simulink model "adc_sim"  (R2017a)
settings: Solver=VariableStepAuto  StartTime=0.0  StopTime=1  FixedStep=0.1e-6  RelTol=1e-3
settings Model: Creator=Andrei Purcarus  LastModifiedBy=Andrei Purcarus

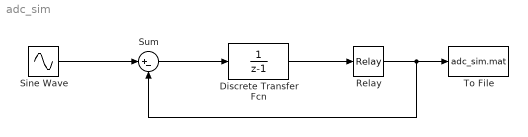
== system adc_sim ==
  Discrete Transfer Fcn : DiscreteTransferFcn  Denominator=[1 -1]  SampleTime=1e-7
  Relay : Relay  OnSwitchValue=0.6  OffSwitchValue=0.6  OnOutputValue=0.84  OffOutputValue=0.36
  Sine Wave : Sin  Amplitude=0.2  Bias=0.6  Frequency=2*pi*20000  SampleTime=0
  Sum : Sum  Inputs=|+-
  To File : ToFile  Filename=adc_sim.mat  SaveFormat=Timeseries
  wires:
  Sine Wave/1 -> Sum/1
  Sum/1 -> Discrete Transfer Fcn/1
  Discrete Transfer Fcn/1 -> Relay/1
  Relay/1 -> To File/1, Sum/2
